simulink model "Exercise_1"  (R2020b)
settings: Solver=VariableStepAuto  StartTime=0.0  StopTime=0.0666666  RelTol=1e-3
libraries: powerlib x10, powerlib_meascontrol x3
settings Model: Creator=ADMIN  LastModifiedBy=macbook
settings SFSimCC: CustomCodeUndefinedFunction=UseInterfaceOnly

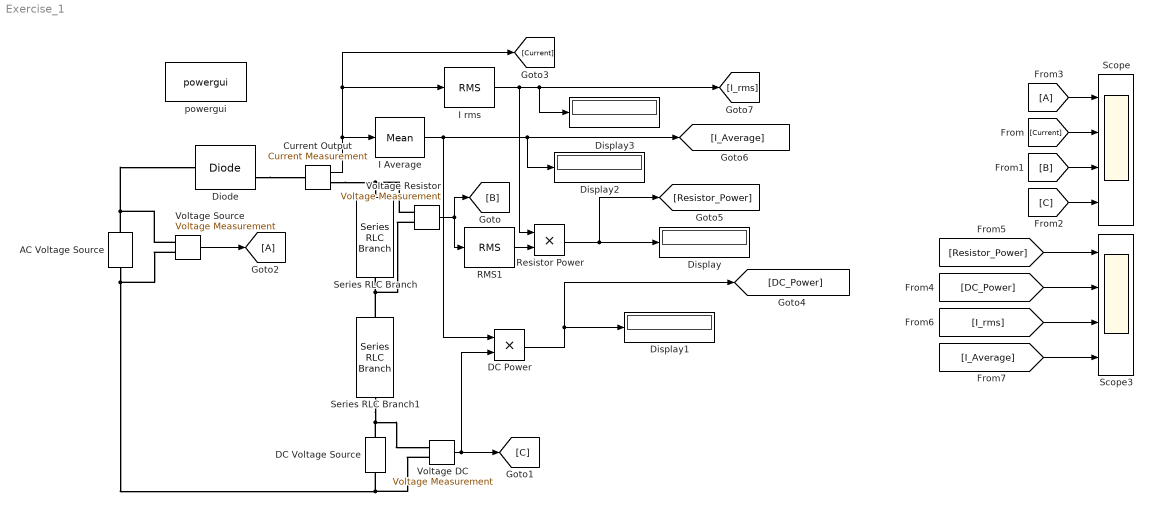
== system Exercise_1 ==
  AC Voltage Source : powerlib/Electrical Sources/AC Voltage Source  Amplitude=169.7  Phase=0  Frequency=60  SampleTime=0  Measurements=None  BusType=swing  Pref=10e3  Qref=0  Qmin=-inf  Qmax=+inf
  Current Output : powerlib/Measurements/Current Measurement  PhasorSimulation=off  OutputType=Complex  PSBequivalent=0
  DC Power : Product
  DC Voltage Source : powerlib/Electrical Sources/DC Voltage Source  Amplitude=48  Measurements=None
  Diode : powerlib/Power Electronics/Diode  Ron=0.001  Lon=0  Vf=0.6  IC=0  UseSnubber=0  Rs=0  Cs=0  Measurements=on
  Display{,1..3} (4 alike) : Display
  I Average : powerlib_meascontrol/Measurements/Mean  Freq=60  Vinit=0  Ts=0
  I rms : powerlib_meascontrol/Measurements/RMS  TrueRMS=on  Freq=60  RMSInit=120  Ts=0
  RMS1 : powerlib_meascontrol/Measurements/RMS  TrueRMS=on  Freq=60  RMSInit=120  Ts=0
  Resistor Power : Product
  Scope : Scope  NumInputPorts=4
  Scope3 : Scope  NumInputPorts=4
  Series RLC Branch : powerlib/Elements/Series RLC Branch  LConnTagsString=__new0  RConnTagsString=__new0  BranchType=R  Resistance=12  Inductance=120e-3  SetiL0=off  InitialCurrent=0  Capacitance=0  Setx0=off  InitialVoltage=0  Measurements=None
  Series RLC Branch1 : powerlib/Elements/Series RLC Branch  LConnTagsString=__new0  RConnTagsString=__new0  BranchType=L  Resistance=1  Inductance=120e-3  SetiL0=off  InitialCurrent=0  Capacitance=1e-6  Setx0=off  InitialVoltage=0  Measurements=None
  Voltage DC : powerlib/Measurements/Voltage Measurement  PhasorSimulation=off  OutputType=Complex  PSBequivalent=0
  Voltage Resistor : powerlib/Measurements/Voltage Measurement  PhasorSimulation=off  OutputType=Complex  PSBequivalent=0
  Voltage Source : powerlib/Measurements/Voltage Measurement  PhasorSimulation=off  OutputType=Complex  PSBequivalent=0
  powergui : powerlib/powergui  Priority=1  SimulationMode=Continuous  SampleTime=50e-6  frequency=60  Iterations=50  frequencyindice=60  Pbase=100e6  ErrMax=1e-4  UnitsV=kV  UnitsW=MW  buscounter=0  FunctionMessages=off  echomessages=off  EnableUseOfTLC=off  CurrentSourceSwitches=off  DisableSnubberDevices=off  DisableRonSwitches=off  DisableVfSwitches=off  DisplayEquations=off  AutomaticDiscreteSolvers=off  SolverType=Tustin/Backward Euler (TBE)  Interpol=off  ExternalGateDelay=off  methode=off  Ts=100  x0status=blocks  SPID=on  SwTol=0  HookPort=off  NonlinearTolerance=0  nMaxIteration=15  ContinueOnMaxIteration=off  RestoreLinks=warning  ResistiveCurrentMeasurement=off  Frange=[0:2:500]  Ylog=off  Xlog=on  ShowGrid=off  save=off  variable=ZData  structure=0  ZoomFFT=off  StartTime=0.0  cycles=1  DisplayStyle=1  fundamental=60  FreqAxis=off  MaxFrequency=1000  frequencyindicesteady=1  RmsSteady=1  display=off
  wires:
  Voltage DC/1 -> [C], DC Power/2
  Voltage Resistor/1 -> RMS1/1, [B]
  DC Power/1 -> [DC_Power], Display1/1
  I rms/1 -> Resistor Power/1, [I_rms], Display3/1
  I Average/1 -> DC Power/1, [I_Average], Display2/1
  Current Output/1 -> I Average/1, [Current], I rms/1
  RMS1/1 -> Resistor Power/2
  Voltage Source/1 -> [A]
  [Current] -> Scope/2
  [C] -> Scope/4
  [A] -> Scope/1
  Resistor Power/1 -> [Resistor_Power], Display/1
  [I_Average] -> Scope3/4
  [I_rms] -> Scope3/3
  [DC_Power] -> Scope3/2
  [Resistor_Power] -> Scope3/1
  [B] -> Scope/3
  connections:
  DC Voltage Source/RConn1 -- Series RLC Branch1/RConn1 -- Voltage DC/LConn1
  AC Voltage Source/RConn1 -- Diode/LConn1 -- Voltage Source/LConn1
  AC Voltage Source/LConn1 -- Voltage DC/LConn2 -- DC Voltage Source/LConn1 -- Voltage Source/LConn2
  Diode/RConn1 -- Current Output/LConn1
  Current Output/RConn1 -- Voltage Resistor/LConn1 -- Series RLC Branch/LConn1
  Voltage Resistor/LConn2 -- Series RLC Branch1/LConn1 -- Series RLC Branch/RConn1
